simulink model "simulation_part_reduced_system_without_fault"  (R2021b)
settings: Solver=ode23t  StartTime=0.0  StopTime=0.2  MaxStep=5e-5  RelTol=1e-3  AbsTol=1e-2
values from neighbouring files (symbols this model uses):
  A = [-753.982236862 0 0 0 0 0 0 0 0 0 0 0 ... (2401 elements, 49x49)]    [A_part.mat]    (also in obtain_original_state_space_matrices.m = test.A; obtain_state_space_matrices.m = test.A; obtain_state_space_matrizes.m = test.A)
  B = [0 0 0 0 0 60.3185789489 -1.14155297593e-39 0 0 0 0 0 ... (147 elements, 49x3)]    [B_part.mat]    (also in obtain_original_state_space_matrices.m = test.B; obtain_state_space_matrices.m = test.B; obtain_state_space_matrizes.m = test.B)
  C = [0 0 0 0 0 0 0 2.79621972711e-07 1.06589466424e-06 8.44094022506e-07 0.0541148976255 0.00859810960201 ... (637 elements, 13x49)]    [C_part.mat]    (also in obtain_original_state_space_matrices.m = test.C; obtain_state_space_matrices.m = test.C; obtain_state_space_matrizes.m = test.C)
  D = [0 0 0 0 0 0 0 0 0 0 0 0 ... (39 elements, 13x3)]    [D_part.mat]    (also in obtain_original_state_space_matrices.m = test.D; obtain_state_space_matrices.m = test.D; obtain_state_space_matrizes.m = test.D)
  initial_states = test.x0    [obtain_original_state_space_matrices.m]    (also in obtain_state_space_matrices.m; obtain_state_space_matrizes.m)
undefined symbols (not defined in the file or in its folder): A_svdkrylov, B_svdkrylov, C_svdkrylov, D_svdkrylov, initial_states_svdkrylov
libraries: spsThreePhaseProgrammableVoltageSourceLib x2, spsThreePhaseVIMeasurementLib x2, spsGroundLib x2, spspowerguiLib x1
settings Model: Creator=The MathWorks, Inc.  LastModifiedBy=amparogonzalezcastano
settings SolverCC: AutoScaleAbsTol=off  AlgebraicLoopSolver=TrustRegion
settings DataIOCC: Decimation=10  SaveFinalState=on  SaveFormat=Array  SaveOutput=off  ReturnWorkspaceOutputs=off  SignalLoggingName=sigsOut
settings OptimizationCC: BlockReduction=off  BooleanDataType=off  ExpressionDepthLimit=2147483647  InitFltsAndDblsToZero=on  LifeSpan=inf
settings DebuggingCC: UnderspecifiedInitializationDetection=Classic  MergeDetectMultiDrivingBlocksExec=none  CheckExecutionContextPreStartOutputMsg=on  SignalResolutionControl=TryResolveAllWithWarning  MultiTaskDSMMsg=warning  MultiTaskCondExecSysMsg=none  SigSpecEnsureSampleTimeMsg=none  FcnCallInpInsideContextMsg=warning  UnconnectedInputMsg=none  UnconnectedOutputMsg=none  StateNameClashWarn=warning  SFUnexpectedBacktrackingDiag=warning  SFNoUnconditionalDefaultTransitionDiag=warning  SFExecutionAtInitializationDiag=none  SFMachineParentedDataDiag=warning  ArithmeticOperatorsInVariantConditions=warning
settings HardwareCC: ProdBitPerPointer=32  ProdBitPerSizeT=32  ProdBitPerPtrDiffT=32  ProdLargestAtomicFloat=None  ProdIntDivRoundTo=Undefined  ProdEndianess=Unspecified  ProdWordSize=32  ProdHWDeviceType=Specified  TargetUnknown=on
settings ModelReferenceCC: PropagateSignalLabelsOutOfModel=off
settings SFSimCC: SimUseLocalCustomCode=off  CustomCodeUndefinedFunction=UseInterfaceOnly
settings RTWCC: RTWUseLocalCustomCode=off
settings CodeAppCC: StateflowObjectComments=on
settings GRTTargetCC: TargetLangStandard=C89/C90 (ANSI)  CombineOutputUpdateFcns=off  GRTInterface=on
settings ConfigComp: CovMetricSettings=dw  CovSaveCumulativeToWorkspaceVar=on  CovSaveSingleToWorkspaceVar=on  CovExternalEMLEnable=off  CovSFcnEnable=off
settings SimscapeCC: SimscapeNormalizeSystem=off

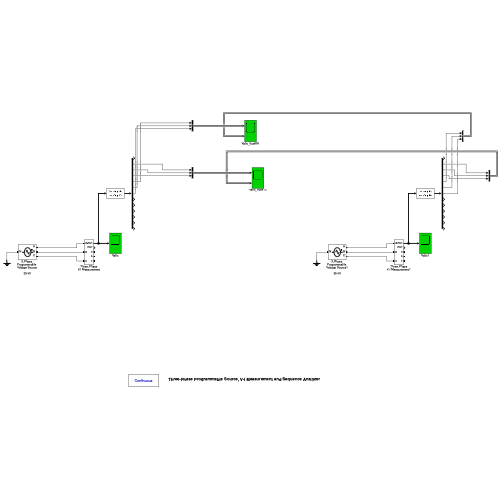
[thumbnail: Simulink's stored preview of the top-level diagram]
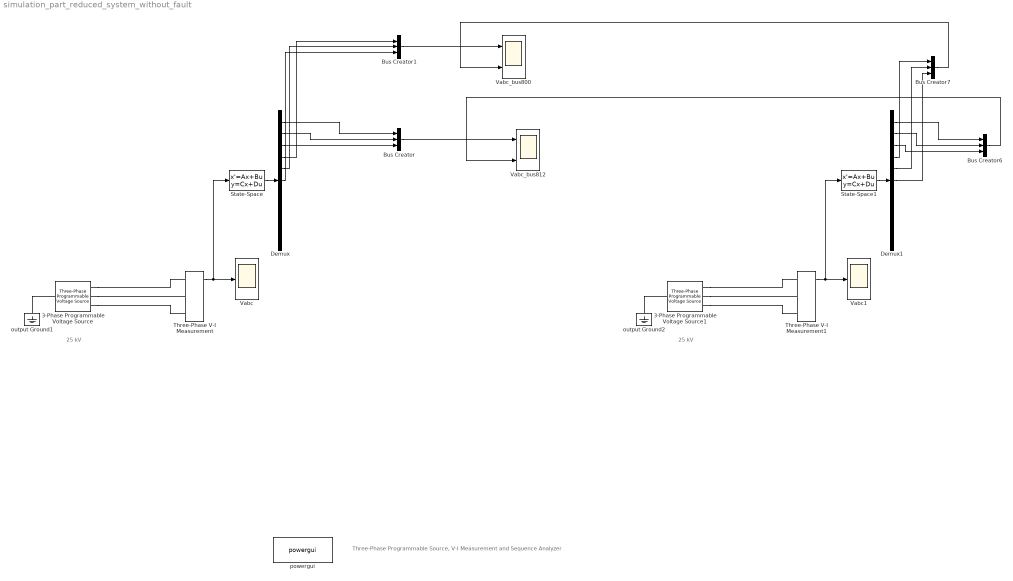
== system simulation_part_reduced_system_without_fault ==
  note: Three-Phase Programmable Source, V-I Measurement and Sequence Analyzer
  note: 25 kV
  note: 25 kV
  3-Phase Programmable Voltage Source : spsThreePhaseProgrammableVoltageSourceLib/Three-Phase Programmable Voltage Source  PositiveSequence="[25e3 0  60]"  VariationEntity=Amplitude  VariationType=Step  VariationTypeAlt=Step  VariationStep=0.5  VariationRate=10  VariationMagnitude=0.3  VariationFrequency=2  VariationTiming=[0 0.5]  VariationPhaseA=off  Amplitudes=[1 0.8 1.2 1.0]  TimeValues=[0 0.1 0.15 0.2]  HarmonicGeneration=off  HarmonicA=[5 0.08 -45 2]  HarmonicB=[2 0 0 2]  Timing="[0.1  1]"  BusType=swing  Pref=0  Qref=0  Qmin=-inf  Qmax=inf
  3-Phase Programmable Voltage Source1 : spsThreePhaseProgrammableVoltageSourceLib/Three-Phase Programmable Voltage Source  PositiveSequence="[25e3 0  60]"  VariationEntity=Amplitude  VariationType=Step  VariationTypeAlt=Step  VariationStep=0.5  VariationRate=10  VariationMagnitude=0.3  VariationFrequency=2  VariationTiming=[0 0.5]  VariationPhaseA=off  Amplitudes=[1 0.8 1.2 1.0]  TimeValues=[0 0.1 0.15 0.2]  HarmonicGeneration=off  HarmonicA=[5 0.08 -45 2]  HarmonicB=[2 0 0 2]  Timing="[0.1  1]"  BusType=swing  Pref=0  Qref=0  Qmin=-inf  Qmax=inf
  Bus Creator{,1,6..7} (4 alike) : BusCreator  Inputs=3
  Demux : Demux  Outputs=13
  Demux1 : Demux  Outputs=13
  State-Space : StateSpace  A=A  B=B  C=C  D=D  InitialCondition=initial_states  AllowTunableDMatrix=on
  State-Space1 : StateSpace  A=A_svdkrylov  B=B_svdkrylov  C=C_svdkrylov  D=D_svdkrylov  InitialCondition=initial_states_svdkrylov  AllowTunableDMatrix=on
  Three-Phase V-I Measurement : spsThreePhaseVIMeasurementLib/Three-Phase V-I Measurement  VoltageMeasurement=phase-to-ground  SetLabelV=off  LabelV=V1  Vpu=off  VpuLL=off  CurrentMeasurement=yes  SetLabelI=off  LabelI=I1  Ipu=off  Pbase=100e6  Vbase=25e3  OutputType=Magnitude  PhasorSimulation=off  PSBequivalent=0
  Three-Phase V-I Measurement1 : spsThreePhaseVIMeasurementLib/Three-Phase V-I Measurement  VoltageMeasurement=phase-to-ground  SetLabelV=off  LabelV=V1  Vpu=off  VpuLL=off  CurrentMeasurement=yes  SetLabelI=off  LabelI=I1  Ipu=off  Pbase=100e6  Vbase=25e3  OutputType=Magnitude  PhasorSimulation=off  PSBequivalent=0
  Vabc : Scope
  Vabc1 : Scope
  Vabc_bus800 : Scope  NumInputPorts=2
  Vabc_bus812 : Scope  NumInputPorts=2
  output Ground1 : spsGroundLib/Ground  LConnTagsString=a
  output Ground2 : spsGroundLib/Ground  LConnTagsString=a
  powergui : spspowerguiLib/powergui  Priority=2  SimulationMode=Continuous  SampleTime=10e-6  frequency=60  Iterations=50  frequencyindice=60  Pbase=100e6  ErrMax=1e-4  UnitsV=kV  UnitsW=MW  buscounter=0  FunctionMessages=off  echomessages=off  EnableUseOfTLC=off  CurrentSourceSwitches=off  DisableSnubberDevices=off  DisableRonSwitches=off  DisableVfSwitches=off  DisplayEquations=off  AutomaticDiscreteSolvers=off  SolverType=Tustin/Backward Euler (TBE)  Interpol=off  ExternalGateDelay=off  methode=off  Ts=0  x0status=blocks  SPID=off  SwTol=0  HookPort=off  NonlinearTolerance=1e-1  nMaxIteration=100  ContinueOnMaxIteration=off  RestoreLinks=warning  ResistiveCurrentMeasurement=off  Frange=[0:2:500]  Ylog=off  Xlog=off  ShowGrid=off  save=off  variable=ZData  structure=0  ZoomFFT=on  StartTime=0.0  cycles=1  DisplayStyle=off  fundamental=60  FreqAxis=off  MaxFrequency=1000  frequencyindicesteady=1  RmsSteady=1  display=off
  wires:
  Three-Phase V-I Measurement/1 -> Vabc/1, State-Space/1
  State-Space/1 -> Demux/1
  State-Space1/1 -> Demux1/1
  Three-Phase V-I Measurement1/1 -> Vabc1/1, State-Space1/1
  Bus Creator1/1 -> Vabc_bus800/1
  Bus Creator/1 -> Vabc_bus812/1
  Bus Creator7/1 -> Vabc_bus800/2
  Bus Creator6/1 -> Vabc_bus812/2
  Demux/2 -> Bus Creator/1
  Demux/3 -> Bus Creator/2
  Demux/4 -> Bus Creator/3
  Demux1/2 -> Bus Creator6/1
  Demux1/3 -> Bus Creator6/2
  Demux1/4 -> Bus Creator6/3
  Demux/5 -> Bus Creator1/1
  Demux/6 -> Bus Creator1/2
  Demux/7 -> Bus Creator1/3
  Demux1/5 -> Bus Creator7/1
  Demux1/6 -> Bus Creator7/2
  Demux1/7 -> Bus Creator7/3
  connections:
  3-Phase Programmable Voltage Source/RConn1 -- Three-Phase V-I Measurement/LConn1
  3-Phase Programmable Voltage Source/RConn2 -- Three-Phase V-I Measurement/LConn2
  3-Phase Programmable Voltage Source/RConn3 -- Three-Phase V-I Measurement/LConn3
  output Ground1/LConn1 -- 3-Phase Programmable Voltage Source/LConn1
  3-Phase Programmable Voltage Source1/RConn2 -- Three-Phase V-I Measurement1/LConn2
  3-Phase Programmable Voltage Source1/RConn1 -- Three-Phase V-I Measurement1/LConn1
  3-Phase Programmable Voltage Source1/RConn3 -- Three-Phase V-I Measurement1/LConn3
  output Ground2/LConn1 -- 3-Phase Programmable Voltage Source1/LConn1
